simulink model "test"  (R2015a)
settings: Solver=ode45  StartTime=0.0  StopTime=10.0  RelTol=1e-3
values from neighbouring files (symbols this model uses):
  K = place(A,B',p)    [discretizareN.m]    (also in statefb.m = place(A2,B2',p))
settings Model: Creator=asus  LastModifiedBy=asus

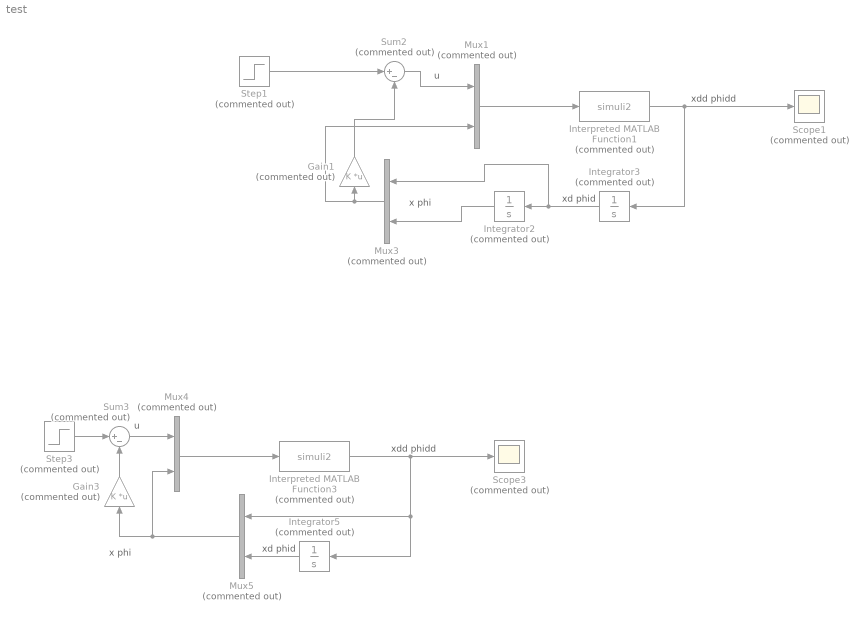
== system test ==
  note: x phi
  note: xd phid
  note: xdd phidd
  note: u
  note: x phi
  note: xd phid
  note: xdd phidd
  note: u
  Gain1 : Gain  Commented=on  Gain=K  Multiplication=Matrix(K*u)
  Gain3 : Gain  Commented=on  Gain=K  Multiplication=Matrix(K*u) (u vector)
  Integrator2 : Integrator  Commented=on  InitialCondition=[0;0]
  Integrator3 : Integrator  Commented=on  InitialCondition=[0;0]
  Integrator5 : Integrator  Commented=on  InitialCondition=[0;0]
  Interpreted MATLAB Function1 : MATLABFcn  Commented=on  MATLABFcn=simuli2
  Interpreted MATLAB Function3 : MATLABFcn  Commented=on  MATLABFcn=simuli2
  Mux{1,3..5} (4 alike) : Mux  Commented=on  Inputs=2
  Scope1 : Scope  Commented=on
      settings: YMin=-1.75e+06  YMax=500000
  Scope3 : Scope  Commented=on
      settings: SaveName=ScopeData3
  Step1 : Step  Commented=on  Time=2  After=5  SampleTime=0
  Step3 : Step  Commented=on  Time=0  After=0  SampleTime=0
  Sum2 : Sum  Commented=on  Inputs=|+-
  Sum3 : Sum  Commented=on  Inputs=|+-
  wires:
  Mux1/1 -> Interpreted MATLAB Function1/1
  Interpreted MATLAB Function1/1 -> Integrator3/1, Scope1/1
  Step1/1 -> Sum2/1
  Sum2/1 -> Mux1/1
  Gain1/1 -> Sum2/2
  Integrator3/1 -> Mux3/1, Integrator2/1
  Mux3/1 -> Mux1/2, Gain1/1
  Integrator2/1 -> Mux3/2
  Mux4/1 -> Interpreted MATLAB Function3/1
  Interpreted MATLAB Function3/1 -> Integrator5/1, Mux5/1, Scope3/1
  Step3/1 -> Sum3/1
  Gain3/1 -> Sum3/2
  Sum3/1 -> Mux4/1
  Integrator5/1 -> Mux5/2
  Mux5/1 -> Gain3/1, Mux4/2
